simulink model "Modulation"  (R2022b)
settings: Solver=VariableStepAuto  StartTime=0.0  StopTime=20.0  RelTol=1e-3
settings Model: Creator=Sahaj Singh  LastModifiedBy=rosie

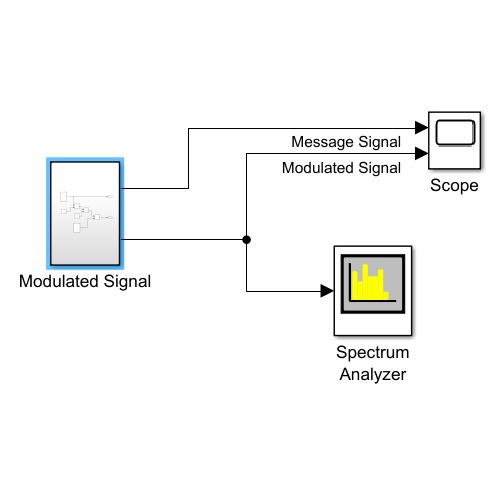
[thumbnail: Simulink's stored preview of the top-level diagram]
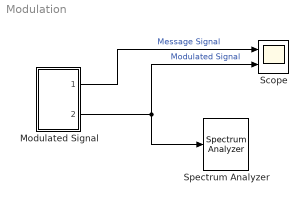
== system Modulation ==
  Modulated Signal : Subsystem
  Scope : Scope  NumInputPorts=2
  Spectrum Analyzer : SpectrumAnalyzer
  wires:
  Modulated Signal/2(" Modulated Signal Output") -> Spectrum Analyzer/1, Scope/2  "Modulated Signal"
  Modulated Signal/1(Message Signal Output) -> Scope/1  "Message Signal"

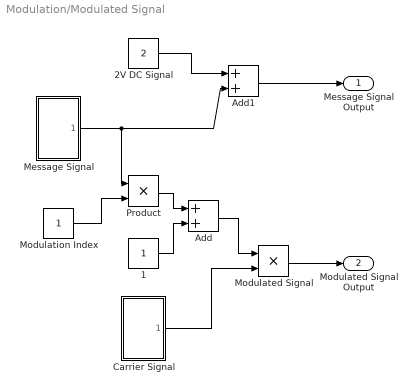
== system Modulation/Modulated Signal ==
  1 : Constant
  2V DC Signal : Constant  Value=2
  Add : Sum
  Add1 : Sum
  Carrier Signal : Subsystem
  Message Signal : Subsystem
  Modulated Signal : Product
  Modulation Index : Constant
  Product : Product
  Message Signal Output : Outport
  " Modulated Signal Output" : Outport  Port=2
  wires:
  Add/1 -> Modulated Signal/1
  Product/1 -> Add/1
  1/1 -> Add/2
  Modulation Index/1 -> Product/2
  Carrier Signal/1(Carrier Signal) -> Modulated Signal/2
  Message Signal/1(Message Signal) -> Add1/2, Product/1
  Modulated Signal/1 -> " Modulated Signal Output"/1
  2V DC Signal/1 -> Add1/1
  Add1/1 -> Message Signal Output/1

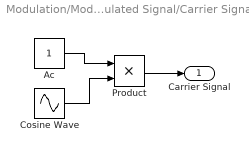
== system Modulation/Modulated Signal/Carrier Signal ==
  Ac : Constant
  Cosine Wave : Sin  Frequency=125663.706137  Phase=1.5708  SampleTime=0.000002
  Product : Product
  Carrier Signal : Outport
  wires:
  Ac/1 -> Product/1
  Cosine Wave/1 -> Product/2
  Product/1 -> Carrier Signal/1

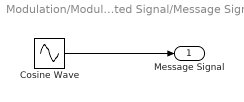
== system Modulation/Modulated Signal/Message Signal ==
  Cosine Wave : Sin  Frequency=12566.370614  Phase=1.5708  SampleTime=0.000002
  Message Signal : Outport
  wires:
  Cosine Wave/1 -> Message Signal/1
